simulink model "Example2"  (R2014a)
settings: Solver=ode45  StartTime=0.0  StopTime=1  RelTol=1e-3
libraries: dspmtrx3 x1
settings Model: Creator=matteo  LastModifiedBy=matteo
settings DebuggingCC: SolverPrmCheckMsg=none

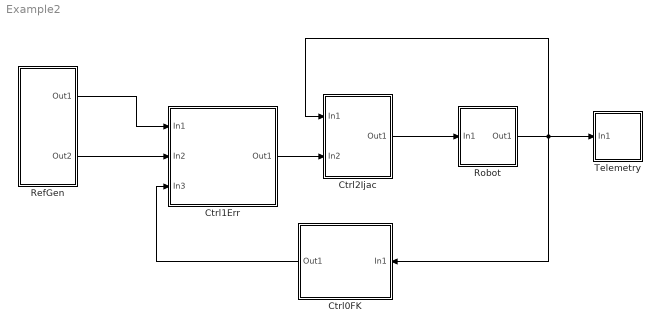
== system Example2 ==
  Ctrl0FK : Subsystem
  Ctrl1Err : Subsystem
  Ctrl2Ijac : Subsystem
  RefGen : Subsystem
  Robot : Subsystem  Tag=plant
  Telemetry : Subsystem  Tag=monitoring
  wires:
  Robot/1(Out1) -> Ctrl0FK/1(In1), Ctrl2Ijac/1(In1), Telemetry/1(In1)
  Ctrl2Ijac/1(Out1) -> Robot/1(In1)
  RefGen/1(Out1) -> Ctrl1Err/1(In1)
  RefGen/2(Out2) -> Ctrl1Err/2(In2)
  Ctrl1Err/1(Out1) -> Ctrl2Ijac/2(In2)
  Ctrl0FK/1(Out1) -> Ctrl1Err/3(In3)

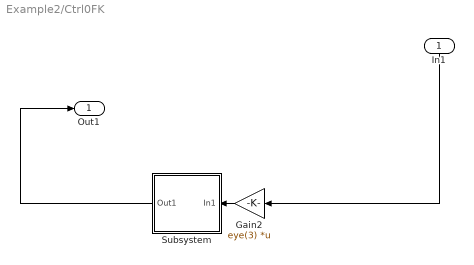
== system Example2/Ctrl0FK ==
  In1 : Inport
  Gain2 : Gain  Gain=eye(3)  Multiplication=Matrix(K*u) (u vector)
  Subsystem : Subsystem
  Out1 : Outport
  wires:
  Gain2/1 -> Subsystem/1(In1)
  Subsystem/1(Out1) -> Out1/1
  In1/1 -> Gain2/1

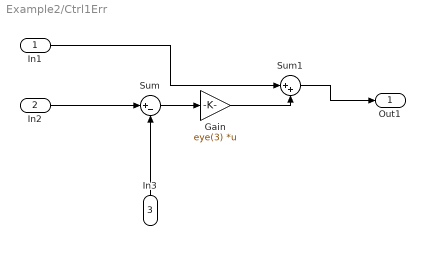
== system Example2/Ctrl1Err ==
  In1 : Inport
  In2 : Inport  Port=2
  In3 : Inport  Port=3
  Gain : Gain  Gain=eye(3)  Multiplication=Matrix(K*u) (u vector)
  Sum : Sum  Inputs=|+-
  Sum1 : Sum  Inputs=|++
  Out1 : Outport
  wires:
  In3/1 -> Sum/2
  In1/1 -> Sum1/1
  In2/1 -> Sum/1
  Sum1/1 -> Out1/1
  Sum/1 -> Gain/1
  Gain/1 -> Sum1/2

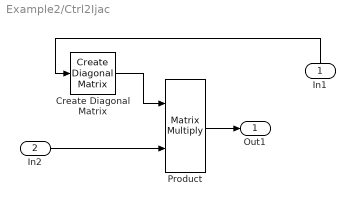
== system Example2/Ctrl2Ijac ==
  In1 : Inport  SampleTime=0.01
  In2 : Inport  Port=2  SampleTime=0.01
  Create Diagonal Matrix : dspmtrx3/Create Diagonal Matrix
  Product : Product  Multiplication=Matrix(*)  SampleTime=0.01
  Out1 : Outport
  wires:
  Product/1 -> Out1/1
  Create Diagonal Matrix/1 -> Product/1
  In1/1 -> Create Diagonal Matrix/1
  In2/1 -> Product/2

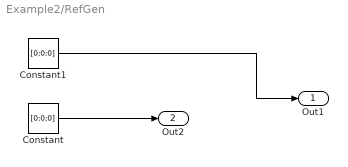
== system Example2/RefGen ==
  Constant : Constant  Value=[0;0;0]
  Constant1 : Constant  Value=[0;0;0]
  Out1 : Outport
  Out2 : Outport  Port=2
  wires:
  Constant1/1 -> Out1/1
  Constant/1 -> Out2/1

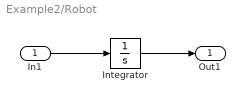
== system Example2/Robot ==
  In1 : Inport
  Integrator : Integrator  InitialCondition=[0;0;0]
  Out1 : Outport
  wires:
  Integrator/1 -> Out1/1
  In1/1 -> Integrator/1

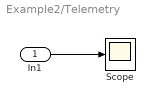
== system Example2/Telemetry ==
  In1 : Inport
  Scope : Scope
  wires:
  In1/1 -> Scope/1

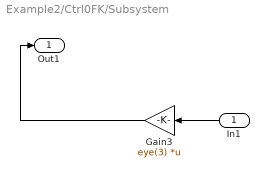
== system Example2/Ctrl0FK/Subsystem ==
  In1 : Inport
  Gain3 : Gain  Gain=eye(3)  Multiplication=Matrix(K*u) (u vector)
  Out1 : Outport
  wires:
  Gain3/1 -> Out1/1
  In1/1 -> Gain3/1
